simulink model "GreenHouseMonitor"  (R2023b)
settings: Solver=FixedStepAuto  StartTime=0.0  StopTime=20  FixedStep=1e-3  RelTol=1e-3
settings Model: Creator=lyndo  LastModifiedBy=lyndo

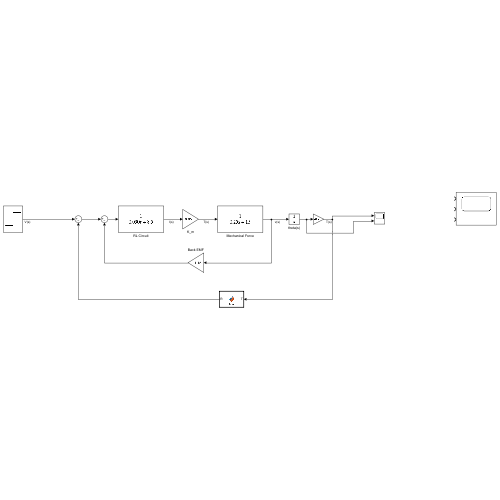
[thumbnail: Simulink's stored preview of the top-level diagram]
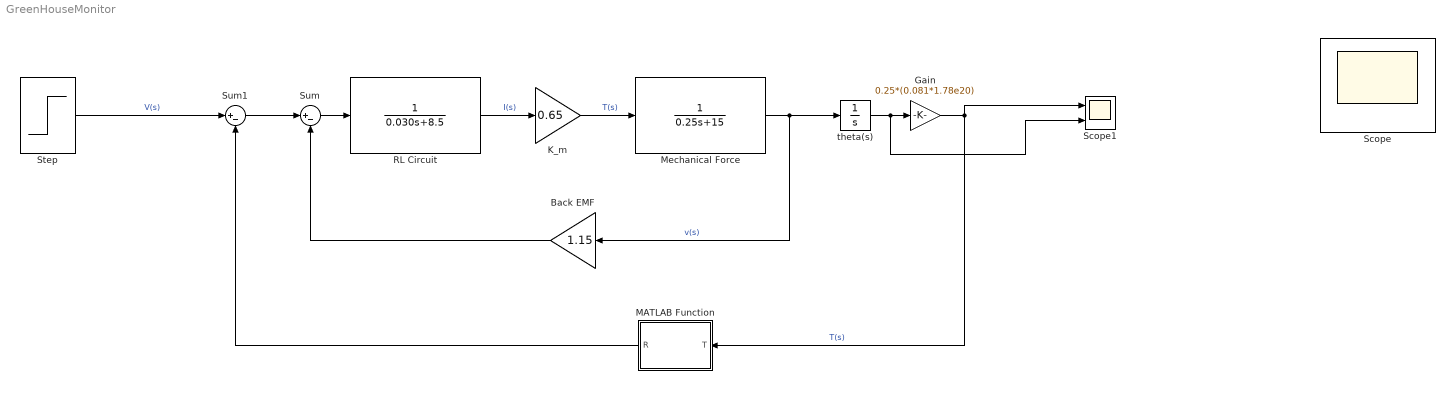
== system GreenHouseMonitor ==
  Back EMF : Gain  Gain=1.15
  Gain : Gain  Gain=0.25*(0.081*1.78e20)
  K_m : Gain  Gain=0.65
  MATLAB Function : MATLAB Function  TreatAsAtomicUnit=on
  Mechanical Force : TransferFcn  Denominator=[0.25 15]
  RL Circuit : TransferFcn  Denominator=[0.030 8.5]
  Scope : Scope  NumInputPorts=3
  Scope1 : Scope  NumInputPorts=2
  Step : Step  Time=0.02  After=12  SampleTime=0.5
  Sum : Sum  Inputs=|+-
  Sum1 : Sum  Inputs=|+-
  theta(s) : Integrator
  wires:
  RL Circuit/1 -> K_m/1  "I(s)"
  K_m/1 -> Mechanical Force/1  "T(s)"
  Mechanical Force/1 -> theta(s)/1, Back EMF/1  "v(s)"
  Sum/1 -> RL Circuit/1
  Back EMF/1 -> Sum/2
  theta(s)/1 -> Scope1/2, Gain/1
  Gain/1 -> MATLAB Function/1(T), Scope1/1  "T(s)"
  Sum1/1 -> Sum/1
  Step/1 -> Sum1/1  "V(s)"
  MATLAB Function/1(R) -> Sum1/2

== matlab function GreenHouseMonitor/MATLAB Function ==
  data: T input; R output
function R = fcn(T)
R_0 = 100;
T_0 = 298.15;
beta = 300

R = R_0*(exp((beta*((1/T)-(1/T_0)))));
